simulink model "simulink_control_b"  (R2023b)
settings: Solver=ode5  StartTime=0.0  StopTime=inf  RelTol=1e-3
values from neighbouring files (symbols this model uses):
  TIME_STEP = 16    [inverted_pendulum_noncart.m]
undefined symbols (not defined in the file or in its folder): accelerometer_sensor, left_rotational_motor, pendulum_sensor, right_rotational_motor
libraries: simulink_extras x1
settings Model: Creator=Harun  LastModifiedBy=Harun
settings RTWCC: GPUComputeCapability=5.0

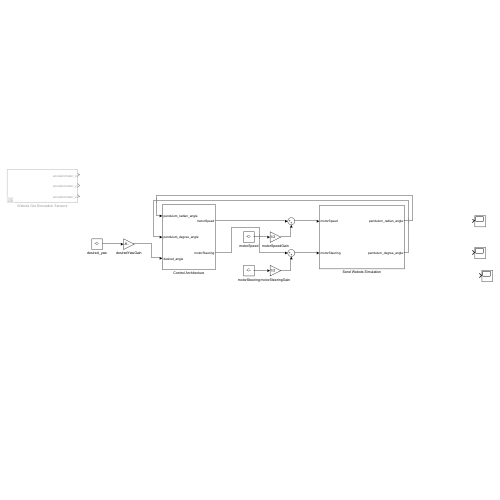
[thumbnail: Simulink's stored preview of the top-level diagram]
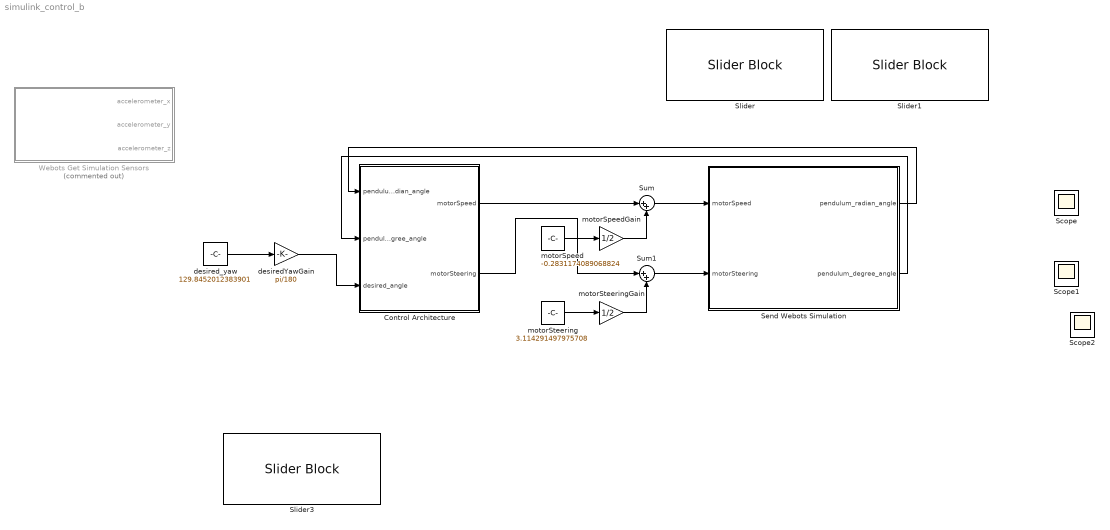
== system simulink_control_b ==
  Control Architecture : Subsystem
  Scope : Scope
  Scope1 : Scope
  Scope2 : Scope
  Send Webots Simulation : Subsystem
  Slider : SliderBlock  ScaleMin=-9.99  ScaleMax=9.99
  Slider1 : SliderBlock  ScaleMin=-9.99  ScaleMax=9.99
  Slider3 : SliderBlock  ScaleMin=-180  ScaleMax=180
  Sum : Sum  Inputs=|++
  Sum1 : Sum  Inputs=|++
  Webots Get Simulation Sensors : Subsystem  Commented=on
  desiredYawGain : Gain  Gain=pi/180
  desired_yaw : Constant  Value=129.8452012383901
  motorSpeed : Constant  Value=-0.2831174089068824
  motorSpeedGain : Gain  Gain=1/2
  motorSteering : Constant  Value=3.114291497975708
  motorSteeringGain : Gain  Gain=1/2
  wires:
  motorSteering/1 -> motorSteeringGain/1
  motorSpeed/1 -> motorSpeedGain/1
  Sum/1 -> Send Webots Simulation/1(motorSpeed)
  Control Architecture/1(motorSpeed) -> Sum/1
  Control Architecture/2(motorSteering) -> Sum1/1
  Sum1/1 -> Send Webots Simulation/2(motorSteering)
  motorSpeedGain/1 -> Sum/2
  motorSteeringGain/1 -> Sum1/2
  desired_yaw/1 -> desiredYawGain/1
  desiredYawGain/1 -> Control Architecture/3(desired_angle)
  Send Webots Simulation/1(pendulum_radian_angle) -> Control Architecture/1(pendulum_radian_angle)
  Send Webots Simulation/2(pendulum_degree_angle) -> Control Architecture/2(pendulum_degree_angle)

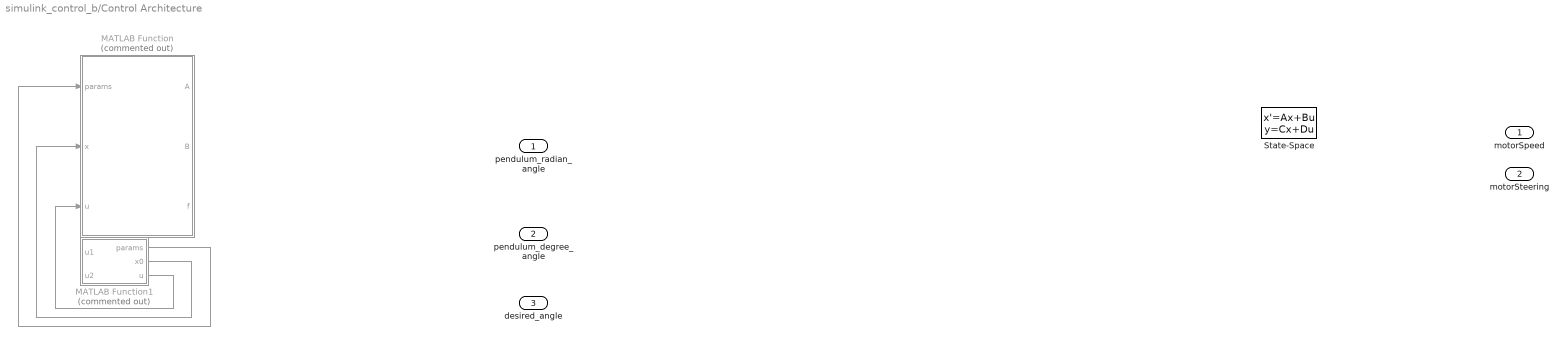
== system simulink_control_b/Control Architecture ==
  pendulum_radian_angle : Inport
  pendulum_degree_angle : Inport  Port=2
  desired_angle : Inport  Port=3
  MATLAB Function : MATLAB Function  Commented=on  TreatAsAtomicUnit=on
  MATLAB Function1 : MATLAB Function  Commented=on  TreatAsAtomicUnit=on
  State-Space : StateSpace  InitialCondition=0
  motorSpeed : Outport
  motorSteering : Outport  Port=2
  wires:
  MATLAB Function1/3(u) -> MATLAB Function/3(u)
  MATLAB Function1/1(params) -> MATLAB Function/1(params)
  MATLAB Function1/2(x0) -> MATLAB Function/2(x)

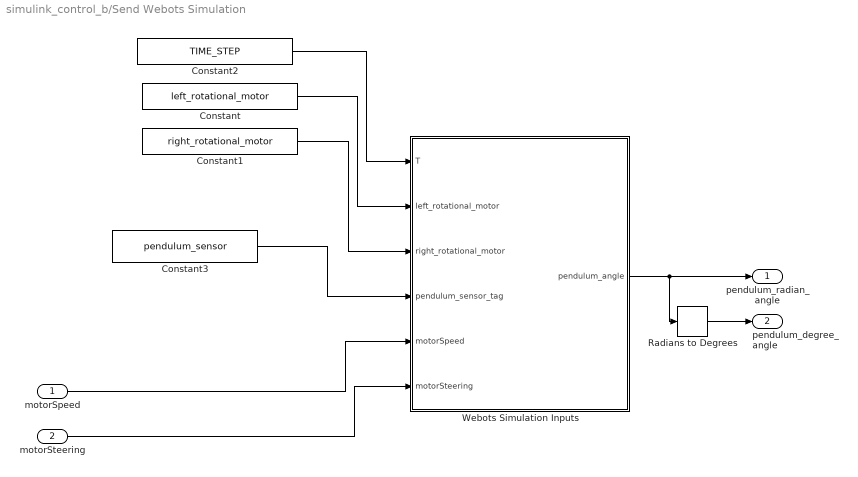
== system simulink_control_b/Send Webots Simulation ==
  motorSpeed : Inport
  motorSteering : Inport  Port=2
  Constant : Constant  Value=left_rotational_motor
  Constant1 : Constant  Value=right_rotational_motor
  Constant2 : Constant  Value=TIME_STEP
  Constant3 : Constant  Value=pendulum_sensor
  Radians to Degrees : simulink_extras/Transformations/Radians to Degrees
  Webots Simulation Inputs : MATLAB Function  TreatAsAtomicUnit=on
  pendulum_radian_angle : Outport
  pendulum_degree_angle : Outport  Port=2
  wires:
  motorSpeed/1 -> Webots Simulation Inputs/5(motorSpeed)
  Constant1/1 -> Webots Simulation Inputs/3(right_rotational_motor)
  Constant2/1 -> Webots Simulation Inputs/1(T)
  Constant/1 -> Webots Simulation Inputs/2(left_rotational_motor)
  Constant3/1 -> Webots Simulation Inputs/4(pendulum_sensor_tag)
  motorSteering/1 -> Webots Simulation Inputs/6(motorSteering)
  Webots Simulation Inputs/1(pendulum_angle) -> Radians to Degrees/1, pendulum_radian_angle/1
  Radians to Degrees/1 -> pendulum_degree_angle/1

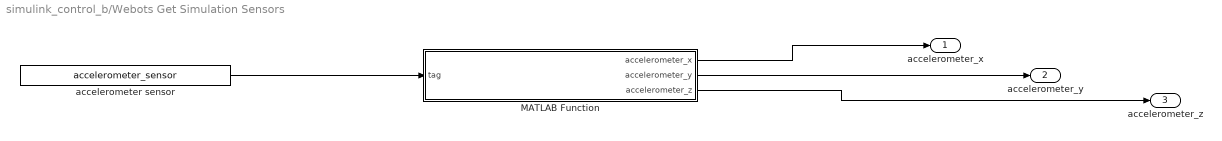
== system simulink_control_b/Webots Get Simulation Sensors ==
  MATLAB Function : MATLAB Function  TreatAsAtomicUnit=on
  accelerometer sensor : Constant  Value=accelerometer_sensor
  accelerometer_x : Outport
  accelerometer_y : Outport  Port=2
  accelerometer_z : Outport  Port=3
  wires:
  accelerometer sensor/1 -> MATLAB Function/1(tag)
  MATLAB Function/1(accelerometer_x) -> accelerometer_x/1
  MATLAB Function/3(accelerometer_z) -> accelerometer_z/1
  MATLAB Function/2(accelerometer_y) -> accelerometer_y/1

== matlab function simulink_control_b/Webots Get Simulation Sensors/MATLAB Function ==
  data: tag input; accelerometer_x output; accelerometer_y output; accelerometer_z output
function [accelerometer_x,accelerometer_y,accelerometer_z] = accelerometer_sensor_get(tag)

period = wb_accelerometer_get_sampling_period(tag)
values = wb_accelerometer_get_values(tag);
accelerometer_x = values(1);
accelerometer_y = values(2);
accelerometer_z = values(3);

== matlab function simulink_control_b/Send Webots Simulation/Webots Simulation Inputs ==
  data: T input; left_rotational_motor input; right_rotational_motor input; pendulum_sensor_tag input; motorSpeed input; motorSteering input; pendulum_angle output
function pendulum_angle =   simulation(T,left_rotational_motor,right_rotational_motor,pendulum_sensor_tag,motorSpeed ...
    ...
    ,motorSteering)

pendulum_angle=0.0
wb_robot_step(T)
wb_motor_set_position(left_rotational_motor, Inf);
wb_motor_set_velocity(left_rotational_motor, motorSpeed-motorSteering);
wb_motor_set_position(right_rotational_motor, Inf);
wb_motor_set_velocity(right_rotational_motor, motorSpeed+motorSteering);

%period = wb_accelerometer_get_sampling_period(accelerometer_tag)
accelerometer_values = wb_position_sensor_get_value(pendulum_sensor_tag);
pendulum_angle = accelerometer_values(1);




end

== matlab function simulink_control_b/Control Architecture/MATLAB Function ==
  data: params input; x input; u input; A output; B output; f output
function [A, B, f] = system_matrices(params, x, u)
    % Parameters
    k1 = params.k1;
    k2 = params.k2;
    m = params.m;
    n = params.n;
    
    A22 = -2 * k2 * (params.Mp * params.R * params.L^2 + params.Mp * params.R^2 * params.L + params.JPt * params.R) / m;
    A23 = -(params.Mp^2 * params.R^2 * params.L^2 * params.g) / m;
    A42 = -2 * k2 / (params.JPt + params.Mp * params.L);
    A43 = (params.Mp * params.g * params.L) / (params.JPt + params.Mp * params.L);
    A66 = -k2 * params.D^2 * params.R / n;

    % A Matrix
    A = [
        0, 1, 0, 0, 0, 0;
        0, A22, A23, 0, 0, 0;
        0, 0, 0, 1, 0, 0;
        0, A42, A43, 0, 0, 0;
        0, 0, 0, 0, 0, 1;
        0, 0, 0, 0, 0, A66;
    ];
    
    % B Matrix
    B21 = -k1 * params.D * params.R / (params.JPt + params.Mp * params.L);
    B62 = k1 * (params.Mp * params.R * params.L^2 + params.Mp * params.R^2 * params.L + params.JPt * params.R) / m;
    B = [
        0, 0;
        B21, 0;
        0, 0;
        0, 0;
        0, 0;
        0, B62;
    ];
    
    % Disturbance Vector f
    f = [0; params.f2; 0; params.f4; 0; params.f6];
end

== matlab function simulink_control_b/Control Architecture/MATLAB Function1 ==
  data: params output; x0 output; u1 input; u2 input; u output
function [params,x0,u] = fcn(u1,u2)
params.N = 100;
params.kt = 0.5;
params.ke = 0.3;
params.Ra = 2.0;
params.Mp = 0.5;
params.g = 9.81;
params.f2 = 0;
params.f4 = 0;
params.f6 = 0;

x0 = [0; 0; 0; 0; 0; 0]; 

u = [0.2; -0.1];
